simulink model "ch7_2nd_Ddelay"  (R2017a)
settings: Solver=ode3  StartTime=0.0  StopTime=1.5  FixedStep=.001  MaxStep=.002  RelTol=1e-3  EnableMultiTasking=on
settings Model: Creator=wintersj  LastModifiedBy=wintersj
settings DataIOCC: LimitDataPoints=on  SaveFormat=Array  SignalLoggingSaveFormat=ModelDataLogs
settings OptimizationCC: ExpressionDepthLimit=2147483647  LifeSpan=inf
settings DebuggingCC: UnderspecifiedInitializationDetection=Classic  MergeDetectMultiDrivingBlocksExec=none  MaxConsecutiveZCsMsg=none  SolverPrmCheckMsg=warning  FcnCallInpInsideContextMsg=warning  StateNameClashWarn=warning  SFUnexpectedBacktrackingDiag=warning  SFNoUnconditionalDefaultTransitionDiag=warning  SFExecutionAtInitializationDiag=none
settings HardwareCC: ProdBitPerPointer=32  ProdBitPerSizeT=32  ProdBitPerPtrDiffT=32  ProdLargestAtomicFloat=None  ProdIntDivRoundTo=Undefined  ProdEndianess=Unspecified  ProdWordSize=32  ProdHWDeviceType=32-bit Generic
settings ModelReferenceCC: PropagateSignalLabelsOutOfModel=off
settings GRTTargetCC: TargetLangStandard=C89/C90 (ANSI)  GeneratePreprocessorConditionals=Disable all  CombineOutputUpdateFcns=off  GRTInterface=on
settings ConfigComp: CovMetricSettings=dw  CovHtmlReporting=on  CovSaveCumulativeToWorkspaceVar=on  CovSaveSingleToWorkspaceVar=on  CovExternalEMLEnable=off

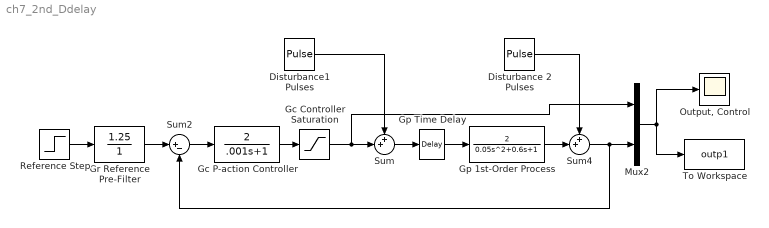
== system ch7_2nd_Ddelay ==
  Disturbance 2 Pulses : DiscretePulseGenerator  PulseType=Time based  Amplitude=0.1  Period=0.4  PulseWidth=50  PhaseDelay=1
  Disturbance1 Pulses : DiscretePulseGenerator  PulseType=Time based  Amplitude=0.1  Period=0.2  PulseWidth=50  PhaseDelay=1.1
  Gc P-action Controller : TransferFcn  Numerator=[0 2]  Denominator=[.001 1]
  Gc Controller Saturation : Saturate  UpperLimit=20  LowerLimit=-20  LinearizeAsGain=off
  "Gp 1st-Order Process " : TransferFcn  Numerator=[2]  Denominator=[0.05 0.6 1]
  Gp Time Delay : TransportDelay  DelayTime=0.1
  Gr Reference Pre-Filter : TransferFcn  Numerator=[1.25]  Denominator=[1]
  Mux2 : Mux  Inputs=2
  "Output, Control" : Scope
  Reference Step : Step  Time=0.4  Before=1  After=5  SampleTime=0
  Sum : Sum  Inputs=++|
  Sum2 : Sum  Inputs=|+-
  Sum4 : Sum  Inputs=++|
  To Workspace : ToWorkspace  VariableName=outp1  SampleTime=-1
  wires:
  Sum2/1 -> Gc P-action Controller/1
  Gc Controller Saturation/1 -> Mux2/1, Sum/2
  "Gp 1st-Order Process "/1 -> Sum4/2
  Sum4/1 -> Sum2/2, Mux2/2
  Mux2/1 -> To Workspace/1, "Output, Control"/1
  Disturbance1 Pulses/1 -> Sum/1
  Disturbance 2 Pulses/1 -> Sum4/1
  Gc P-action Controller/1 -> Gc Controller Saturation/1
  Sum/1 -> Gp Time Delay/1
  Gp Time Delay/1 -> "Gp 1st-Order Process "/1
  Gr Reference Pre-Filter/1 -> Sum2/1
  Reference Step/1 -> Gr Reference Pre-Filter/1
